simulink model "motor_ppd"  (R2021a)
settings: Solver=VariableStepAuto  StartTime=0.0  StopTime=1/0  RelTol=1e-3
libraries: spsThreePhaseProgrammableVoltageSourceLib x1, spsAsynchronousMachineSIUnitsLib x1, simulink x1, spsGroundLib x1, spsThreePhaseVIMeasurementLib x1, dspnetwork x1, spsVoltageMeasurementLib x1, spspowerguiLib x1
settings Model: Creator=user  LastModifiedBy=user

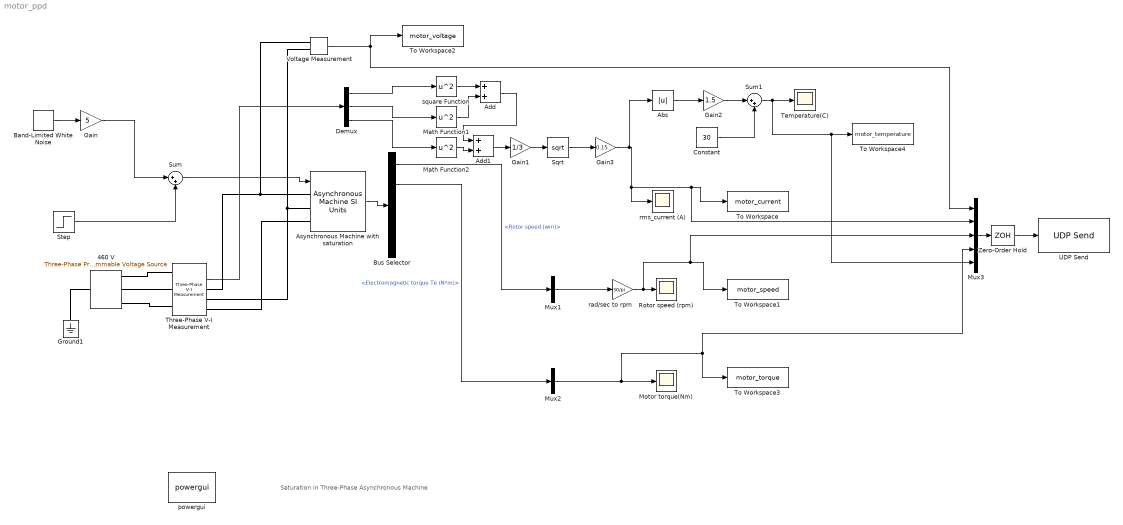
== system motor_ppd ==
  note: Saturation in Three-Phase Asynchronous Machine
  460 V : spsThreePhaseProgrammableVoltageSourceLib/Three-Phase Programmable Voltage Source  PositiveSequence="[460  0 60]"  VariationEntity=None  VariationType=Step  VariationTypeAlt=Step  VariationStep=0.5  VariationRate=10  VariationMagnitude=0.3  VariationFrequency=2  VariationTiming=[1 2]  VariationPhaseA=off  Amplitudes=[1 0.8 1.2 1.0]  TimeValues=[0 0.1 0.15 0.2]  HarmonicGeneration=off  HarmonicA=[3 0.2 -25 0]  HarmonicB=[2 0.15 35 2]  Timing="[0.05  3]"  BusType=swing  Pref=0  Qref=0  Qmin=-inf  Qmax=inf
  Abs : Abs
  Add : Sum
  Add1 : Sum
  Asynchronous Machine with saturation : spsAsynchronousMachineSIUnitsLib/Asynchronous Machine SI Units  RotorType=Squirrel-cage  PresetModel=No  MechanicalLoad=Torque Tm  ShowDetailedParameters=on  ReferenceFrame=Rotor  Units=SI  MeasurementBus=off  NominalParameters=[37300 460 60]  VoltageRatio=1  Stator=[0.087 0.302/377]  Rotor=[0.228 0.302/377]  Cage1=[ 0.022 0.226/377]  Cage2=[ 0.022 0.226/377]  Lm=13.08/377  Mechanical=[1.662 0 2]  PolePairs=2  InitialConditions="[ 1,0   0,0,0   0,0,0 ]"  SimulateSaturation=on  Saturation=[9.9249,19.6672,38.0377,51.3988,69.2824,105.1337,152.5532,214.2421,302;230, 322, 414, 460, 506, 552, 598, 644, 690]  LoadFlowParameters=0  TsPowergui=0  TsBlock=-1  IterativeModel=Trapezoidal non iterative  IterativeDiscreteModel=Trapezoidal non iterative  Pmec=0
  Band-Limited White Noise : simulink/Sources/Band-Limited White Noise  Cov=[0.1]  Ts=0.01  seed=[23341]
  Bus Selector : BusSelector  OutputSignals=Mechanical.Rotor speed (wm),Mechanical.Electromagnetic torque Te (N*m),Stator measurements.Stator current is_a (A),Stator measurements.Stator current is_b (A),Stator measurements.Stator current is_c (A)
  Constant : Constant  Value=30
  Demux : Demux  Outputs=3
  Gain : Gain  Gain=5
  Gain1 : Gain  Gain=1/3
  Gain2 : Gain  Gain=1.5
  Gain3 : Gain  Gain=0.15
  Ground1 : spsGroundLib/Ground  LConnTagsString=a
  Math Function1 : Math  Operator=square  SaturateOnIntegerOverflow=on
  Math Function2 : Math  Operator=square  SaturateOnIntegerOverflow=on
  Motor torque(Nm) : Scope
  Mux1 : Mux  Inputs=1
  Mux2 : Mux  Inputs=1
  Mux3 : Mux  Inputs=5
  Rotor speed (rpm) : Scope
  Sqrt : Sqrt  SaturateOnIntegerOverflow=on
  Step : Step  Time=2  Before=5  After=15  SampleTime=0
  Sum : Sum  Inputs=|++
  Sum1 : Sum  Inputs=|++
  Temperature(C) : Scope
  Three-Phase V-I Measurement : spsThreePhaseVIMeasurementLib/Three-Phase V-I Measurement  VoltageMeasurement=phase-to-ground  SetLabelV=off  LabelV=Vabc  Vpu=off  VpuLL=off  CurrentMeasurement=yes  SetLabelI=off  LabelI=Iabc  Ipu=off  Pbase=100e6  Vbase=500e3  OutputType=Complex  PhasorSimulation=off  PSBequivalent=0
  To Workspace : ToWorkspace  VariableName=motor_current  SampleTime=-1
  To Workspace1 : ToWorkspace  VariableName=motor_speed  SampleTime=-1
  To Workspace2 : ToWorkspace  VariableName=motor_voltage  SampleTime=-1
  To Workspace3 : ToWorkspace  VariableName=motor_torque  SampleTime=-1
  To Workspace4 : ToWorkspace  VariableName=motor_temperature  SampleTime=-1
  UDP Send : dspnetwork/UDP Send  remoteURL='127.0.0.1'  remotePort=5005  localURL='0.0.0.0'  localPortSource=Automatically determine  localPort=-1  sendBufferSize=8192  sampletime=-1  blockPlatform=[]  separateLengthPort=0
  Voltage Measurement : spsVoltageMeasurementLib/Voltage Measurement  PhasorSimulation=off  OutputType=Complex  PSBequivalent=0
  Zero-Order Hold : ZeroOrderHold  SampleTime=5
  powergui : spspowerguiLib/powergui  Priority=2  SimulationMode=Continuous  SampleTime=0  frequency=60  Iterations=50  frequencyindice=60  Pbase=100e6  ErrMax=1e-4  UnitsV=kV  UnitsW=MW  buscounter=0  FunctionMessages=off  echomessages=off  EnableUseOfTLC=off  CurrentSourceSwitches=off  DisableSnubberDevices=off  DisableRonSwitches=off  DisableVfSwitches=off  DisplayEquations=off  AutomaticDiscreteSolvers=off  SolverType=Tustin  Interpol=off  ExternalGateDelay=off  methode=off  Ts=0  x0status=blocks  SPID=off  SwTol=0  HookPort=off  NonlinearTolerance=1e-4  nMaxIteration=100  ContinueOnMaxIteration=off  RestoreLinks=warning  ResistiveCurrentMeasurement=off  Frange=[0:2:500]  Ylog=off  Xlog=on  ShowGrid=off  save=off  variable=ZData  structure=0  ZoomFFT=on  StartTime=0.0  cycles=1  DisplayStyle=1  fundamental=60  FreqAxis=off  MaxFrequency=1000  frequencyindicesteady=1  RmsSteady=1  display=off
  rad/sec to rpm : Gain  Gain=30/pi
  rms_current (A) : Scope
  square Function : Math  Operator=square  SaturateOnIntegerOverflow=on
  wires:
  Mux1/1 -> rad/sec to rpm/1
  rad/sec to rpm/1 -> Mux3/3, To Workspace1/1, Rotor speed (rpm)/1
  Asynchronous Machine with saturation/1 -> Bus Selector/1
  Bus Selector/1 -> Mux1/1  "<Rotor speed (wm)>"
  Voltage Measurement/1 -> Mux3/1, To Workspace2/1
  Band-Limited White Noise/1 -> Gain/1
  Gain/1 -> Sum/1
  Step/1 -> Sum/2
  Bus Selector/2 -> Mux2/1  "<Electromagnetic torque Te (N*m)>"
  Mux2/1 -> To Workspace3/1, Mux3/4, Motor torque(Nm)/1
  Mux3/1 -> Zero-Order Hold/1
  Zero-Order Hold/1 -> UDP Send/1
  square Function/1 -> Add/1
  Math Function1/1 -> Add/2
  Add/1 -> Add1/1
  Math Function2/1 -> Add1/2
  Add1/1 -> Gain1/1
  Gain1/1 -> Sqrt/1
  Gain3/1 -> Abs/1, Mux3/2, To Workspace/1, rms_current (A)/1
  Abs/1 -> Gain2/1
  Gain2/1 -> Sum1/1
  Constant/1 -> Sum1/2
  Sum1/1 -> Mux3/5, To Workspace4/1, Temperature(C)/1
  Three-Phase V-I Measurement/2 -> Demux/1
  Demux/1 -> square Function/1
  Demux/2 -> Math Function1/1
  Demux/3 -> Math Function2/1
  Sqrt/1 -> Gain3/1
  Sum/1 -> Asynchronous Machine with saturation/1
  connections:
  Voltage Measurement/LConn1 -- Asynchronous Machine with saturation/LConn1 -- Three-Phase V-I Measurement/RConn1
  Voltage Measurement/LConn2 -- Three-Phase V-I Measurement/RConn2 -- Asynchronous Machine with saturation/LConn2
  Ground1/LConn1 -- 460 V/LConn1
  460 V/RConn2 -- Three-Phase V-I Measurement/LConn2
  460 V/RConn3 -- Three-Phase V-I Measurement/LConn3
  Three-Phase V-I Measurement/RConn3 -- Asynchronous Machine with saturation/LConn3
  460 V/RConn1 -- Three-Phase V-I Measurement/LConn1
